simulink model "successPIDClosedLoop20picont"  (R2023b)
settings: Solver=FixedStepAuto  StartTime=0.0  StopTime=inf  RelTol=1e-3  EnableMultiTasking=on
libraries: arduinolib x5, simulink x1, arduinosensorlib x1, slpidlib x1
(part 3 of 3)

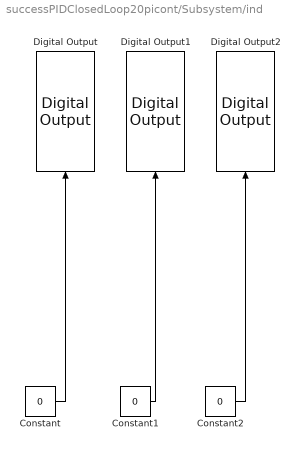
== system successPIDClosedLoop20picont/Subsystem/ind ==
  Constant : Constant  Value=0  SampleTime=0.001
  Constant1 : Constant  Value=0  SampleTime=0.001
  Constant2 : Constant  Value=0  SampleTime=0.001
  Digital Output : arduinolib/Digital Output  pinNumber=7  Direction=output  blockPlatform=arduino
  Digital Output1 : arduinolib/Digital Output  pinNumber=8  Direction=output  blockPlatform=arduino
  Digital Output2 : arduinolib/Digital Output  pinNumber=9  Direction=output  blockPlatform=arduino
  wires:
  Constant2/1 -> Digital Output2/1
  Constant/1 -> Digital Output/1
  Constant1/1 -> Digital Output1/1
